simulink model "AirCraft_Fuel_Distribution"  (R2023b)
settings: Solver=VariableStepAuto  StartTime=0.0  StopTime=8000  MaxStep=10  RelTol=1e-04  AbsTol=1e-04
undefined symbols (not defined in the file): cutoff_time_const, mover_time_constant, opening_max, pump_engine, pump_wing, rho_ref, vol_fuel_min
libraries: fl_lib x52, nesl_utility x33, SimscapeFluids_lib x17, simulink_extras x11, SignalEditorBlockLib x2
(part 1 of 2)
settings Model: Creator=Asus
settings SolverCC: MaxConsecutiveMinStep=4  ZeroCrossAlgorithm=Adaptive  AlgebraicLoopSolver=LineSearch
settings DebuggingCC: AlgebraicLoopMsg=none  IgnoredZcDiagnostic=none  UnconnectedInputMsg=warning  UnconnectedOutputMsg=warning  UnconnectedLineMsg=warning
settings ModelReferenceCC: EnableRefExpFcnMdlSchedulingChecks=on

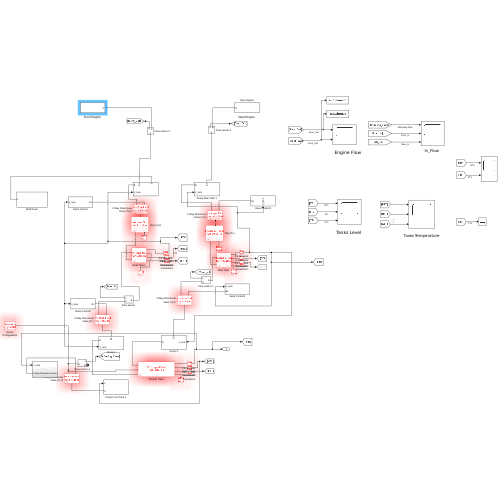
[thumbnail: Simulink's stored preview of the top-level diagram]
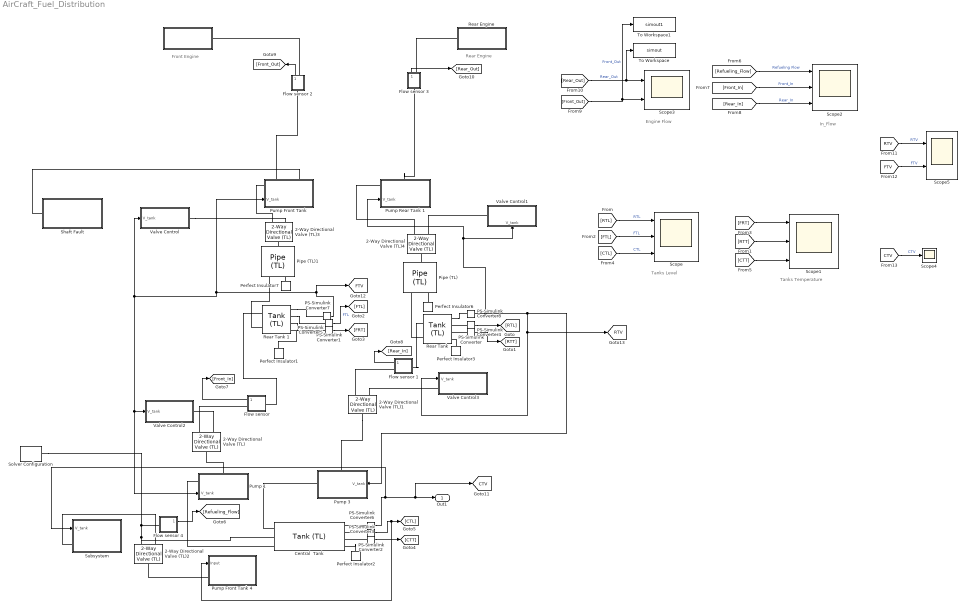
== system AirCraft_Fuel_Distribution ==
  note: Front Engine
  note: Rear Engine
  note: Tanks Temperature
  note: Tanks Level
  note: In_Flow
  note: Engine Flow
  " " : Subsystem
  2-Way Directional Valve (TL) : SimscapeFluids_lib/Thermal Liquid/Valves & Orifices/Directional Control Valves/2-Way Directional Valve (TL)  valve_spec=fluids.thermal_liquid.valves.enum.orifice_spec.linear  opening_max=opening_max m  area_max=area_max m^2  area_leak=1e-10 m^2  smoothing_factor=0.01  opening_TLU=[-.002, 0, .002, .005, .015] m  valve_area_TLU=[1e-09, 2.0352e-07, 4.0736e-05, .00011438, .00034356] m^2  Cd=0.7  Re_c=12  opening_mdot_TLU=[-.002, 0, .002, .005, .015] m  p_diff_TLU=[-.1, .3, .5, .7] MPa  mdot_TLU=[-1e-05, 1.7e-05, 2e-05, 2.6e-05; -.002, .0035, .0045, .0053; -.4, .7, .9, 1.06; -1.13, 1.96, 2.5, 3; -3.45, 6, 7.7, 9.13] kg/s  T_ref_in=293.15 K  p_ref_in=0.101325 MPa  x0=area_max m  area=0.001 m^2  length=0.1 m
      settings: InternalSimscapePortConfiguration="{\"Bottom\":[],\"Left\":[{\"id\":\"A\",\"label\":\"A\",\"type\":\"foundation.thermal_liquid.thermal_liquid\"}],\"Right\":[{\"id\":\"S\",\"label\":\"S\",\"type\":\"input\"},{\"id\":\"B\",\"label\":\"B\",\"type\":\"foundation.thermal_liquid.thermal_liquid\"}],\"Top\":[]}"
  2-Way Directional Valve (TL)1 : SimscapeFluids_lib/Thermal Liquid/Valves & Orifices/Directional Control Valves/2-Way Directional Valve (TL)  valve_spec=fluids.thermal_liquid.valves.enum.orifice_spec.linear  opening_max=opening_max m  area_max=area_max m^2  area_leak=1e-10 m^2  smoothing_factor=0.01  opening_TLU=[-.002, 0, .002, .005, .015] m  valve_area_TLU=[1e-09, 2.0352e-07, 4.0736e-05, .00011438, .00034356] m^2  Cd=0.7  Re_c=12  opening_mdot_TLU=[-.002, 0, .002, .005, .015] m  p_diff_TLU=[-.1, .3, .5, .7] MPa  mdot_TLU=[-1e-05, 1.7e-05, 2e-05, 2.6e-05; -.002, .0035, .0045, .0053; -.4, .7, .9, 1.06; -1.13, 1.96, 2.5, 3; -3.45, 6, 7.7, 9.13] kg/s  T_ref_in=293.15 K  p_ref_in=0.101325 MPa  x0=opening_max m  area=0.001 m^2  length=0.1 m
      settings: InternalSimscapePortConfiguration="{\"Bottom\":[],\"Left\":[{\"id\":\"A\",\"label\":\"A\",\"type\":\"foundation.thermal_liquid.thermal_liquid\"}],\"Right\":[{\"id\":\"S\",\"label\":\"S\",\"type\":\"input\"},{\"id\":\"B\",\"label\":\"B\",\"type\":\"foundation.thermal_liquid.thermal_liquid\"}],\"Top\":[]}"
  2-Way Directional Valve (TL)2 : SimscapeFluids_lib/Thermal Liquid/Valves & Orifices/Directional Control Valves/2-Way Directional Valve (TL)  valve_spec=fluids.thermal_liquid.valves.enum.orifice_spec.linear  opening_max=opening_max m  area_max=area_max m^2  area_leak=1e-10 m^2  smoothing_factor=0.01  opening_TLU=[-.002, 0, .002, .005, .015] m  valve_area_TLU=[1e-09, 2.0352e-07, 4.0736e-05, .00011438, .00034356] m^2  Cd=0.7  Re_c=12  opening_mdot_TLU=[-.002, 0, .002, .005, .015] m  p_diff_TLU=[-.1, .3, .5, .7] MPa  mdot_TLU=[-1e-05, 1.7e-05, 2e-05, 2.6e-05; -.002, .0035, .0045, .0053; -.4, .7, .9, 1.06; -1.13, 1.96, 2.5, 3; -3.45, 6, 7.7, 9.13] kg/s  T_ref_in=293.15 K  p_ref_in=0.101325 MPa  x0=area_max m  area=0.001 m^2  length=0.1 m
      settings: InternalSimscapePortConfiguration="{\"Bottom\":[],\"Left\":[{\"id\":\"A\",\"label\":\"A\",\"type\":\"foundation.thermal_liquid.thermal_liquid\"}],\"Right\":[{\"id\":\"S\",\"label\":\"S\",\"type\":\"input\"},{\"id\":\"B\",\"label\":\"B\",\"type\":\"foundation.thermal_liquid.thermal_liquid\"}],\"Top\":[]}"
  2-Way Directional Valve (TL)3 : SimscapeFluids_lib/Thermal Liquid/Valves & Orifices/Directional Control Valves/2-Way Directional Valve (TL)  valve_spec=fluids.thermal_liquid.valves.enum.orifice_spec.linear  opening_max=opening_max m  area_max=area_max m^2  area_leak=1e-10 m^2  smoothing_factor=0.01  opening_TLU=[-.002, 0, .002, .005, .015] m  valve_area_TLU=[1e-09, 2.0352e-07, 4.0736e-05, .00011438, .00034356] m^2  Cd=0.7  Re_c=12  opening_mdot_TLU=[-.002, 0, .002, .005, .015] m  p_diff_TLU=[-.1, .3, .5, .7] MPa  mdot_TLU=[-1e-05, 1.7e-05, 2e-05, 2.6e-05; -.002, .0035, .0045, .0053; -.4, .7, .9, 1.06; -1.13, 1.96, 2.5, 3; -3.45, 6, 7.7, 9.13] kg/s  T_ref_in=293.15 K  p_ref_in=0.101325 MPa  x0=opening_max m  area=0.001 m^2  length=0.1 m
      settings: InternalSimscapePortConfiguration="{\"Bottom\":[],\"Left\":[{\"id\":\"A\",\"label\":\"A\",\"type\":\"foundation.thermal_liquid.thermal_liquid\"}],\"Right\":[{\"id\":\"S\",\"label\":\"S\",\"type\":\"input\"},{\"id\":\"B\",\"label\":\"B\",\"type\":\"foundation.thermal_liquid.thermal_liquid\"}],\"Top\":[]}"
  2-Way Directional Valve (TL)4 : SimscapeFluids_lib/Thermal Liquid/Valves & Orifices/Directional Control Valves/2-Way Directional Valve (TL)  valve_spec=fluids.thermal_liquid.valves.enum.orifice_spec.linear  opening_max=opening_max m  area_max=area_max m^2  area_leak=1e-10 m^2  smoothing_factor=0.01  opening_TLU=[-.002, 0, .002, .005, .015] m  valve_area_TLU=[1e-09, 2.0352e-07, 4.0736e-05, .00011438, .00034356] m^2  Cd=0.7  Re_c=12  opening_mdot_TLU=[-.002, 0, .002, .005, .015] m  p_diff_TLU=[-.1, .3, .5, .7] MPa  mdot_TLU=[-1e-05, 1.7e-05, 2e-05, 2.6e-05; -.002, .0035, .0045, .0053; -.4, .7, .9, 1.06; -1.13, 1.96, 2.5, 3; -3.45, 6, 7.7, 9.13] kg/s  T_ref_in=293.15 K  p_ref_in=0.101325 MPa  x0=opening_max m  area=0.001 m^2  length=0.1 m
      settings: InternalSimscapePortConfiguration="{\"Bottom\":[],\"Left\":[{\"id\":\"A\",\"label\":\"A\",\"type\":\"foundation.thermal_liquid.thermal_liquid\"}],\"Right\":[{\"id\":\"S\",\"label\":\"S\",\"type\":\"input\"},{\"id\":\"B\",\"label\":\"B\",\"type\":\"foundation.thermal_liquid.thermal_liquid\"}],\"Top\":[]}"
  "Central  Tank " : SimscapeFluids_lib/Thermal Liquid/Tanks & Accumulators/Tank (TL)  pressure_spec=2  tank_pressure=p_tank MPa  max_capacity=384 m^3  volume_spec=2  tank_area=center_tank_level_TLU m^2  level_TLU=center_tank_level_TLU m  volume_TLU=center_tank_volume_TLU m^3  inlet_height=0.1 m  inlet_area=0.01 m^2  g=9.81 m/s^2  level_specify=on  level_priority=High  level=0.5 m  level_nominal_specify=off  level_nominal_unit=m  level_nominal_value=1  volume_specify=on  volume_priority=None  volume=3 m^3  volume_nominal_specify=off  volume_nominal_unit=m^3  volume_nominal_value=1  mass_specify=off  mass_priority=None  mass=5e+3 kg  mass_nominal_specify=off  mass_nominal_unit=kg  mass_nominal_value=1  T_tank_specify=on  T_tank_priority=High  T_tank=T0 K  T_tank_nominal_specify=off  T_tank_nominal_unit=K  T_tank_nominal_value=1  inlet_heights_AB=[.1, 0] m  inlet_areas_AB=[.01, .01] m^2  inlet_heights_ABC=[1e-4, 1e-4, 0] m  inlet_areas_ABC=7e-4 .* ones(1,3) m^2
      settings: InternalSimscapePortConfiguration="{\"Bottom\":[],\"Left\":[{\"id\":\"A\",\"label\":\"A\",\"type\":\"foundation.thermal_liquid.thermal_liquid\"},{\"id\":\"B\",\"label\":\"B\",\"type\":\"foundation.thermal_liquid.thermal_liquid\"},{\"id\":\"C\",\"label\":\"C\",\"type\":\"foundation.thermal_liquid.thermal_liquid\"}],\"Right\":[{\"id\":\"V_out\",\"label\":\"V\",\"type\":\"output\"},{\"id\":\"L_out\",\"label\":\"L\",\"type\":\"output\"},{\"id\":\"T_out\",\"label\":\"T\",\"type\":\"output\"},{\"id\":\"H\",\"label\":\"H\",\"type\":\"foundation.thermal.thermal\"}],\"Top\":[]}"
  "Flow sensor " : Subsystem
      settings: PortSchema="{\"entries\":[{\"content\":{\"sides\":[{\"content\":{\"connectorIds\":[\"Out1\",\"LConn1\"]},\"type\":\"ConnectorPlacement.EquallySpacedRectSide\",\"uuid\":\"5284a614-22fb-4539-b8c2-000aa98607e7\"},{\"content\":{\"connectorIds\":[\"RConn1\"],\"side\":\"RIGHT\"},\"type\":\"ConnectorPlacement.EquallySpacedRectSide\",\"uuid\":\"ab54947e-968b-43fc-9d3b-310523b757f2\"},{\"content\":{\"connectorIds\":[],\"side\":\"TOP\"},\"type\":\"ConnectorPlacement.EquallySpacedRectSide\",\"uuid\":\"346eb7b4-d6d4-447e-a1ee-2e30abc93d9f\"}]},\"type\":\"ConnectorPlacement.EquallySpacedConnector\",\"uuid\":\"c574b111-9014-4fd2-84a0-cd6807004c01\"}],\"packageUris\":[\"http://schema.mathworks.com/mf0/Connector/19700101\"],\"version\":\"1.0\"}"
  Flow sensor 1 : Subsystem
      settings: PortSchema="{\"entries\":[{\"content\":{\"sides\":[{\"content\":{\"connectorIds\":[\"Out1\",\"LConn1\"]},\"type\":\"ConnectorPlacement.EquallySpacedRectSide\",\"uuid\":\"5284a614-22fb-4539-b8c2-000aa98607e7\"},{\"content\":{\"connectorIds\":[\"RConn1\"],\"side\":\"RIGHT\"},\"type\":\"ConnectorPlacement.EquallySpacedRectSide\",\"uuid\":\"ab54947e-968b-43fc-9d3b-310523b757f2\"},{\"content\":{\"connectorIds\":[],\"side\":\"TOP\"},\"type\":\"ConnectorPlacement.EquallySpacedRectSide\",\"uuid\":\"346eb7b4-d6d4-447e-a1ee-2e30abc93d9f\"}]},\"type\":\"ConnectorPlacement.EquallySpacedConnector\",\"uuid\":\"c574b111-9014-4fd2-84a0-cd6807004c01\"}],\"packageUris\":[\"http://schema.mathworks.com/mf0/Connector/19700101\"],\"version\":\"1.0\"}"
  Flow sensor 2 : Subsystem
  Flow sensor 3 : Subsystem
  Flow sensor 4 : Subsystem
  PS-Simulink Converter{,1..8} (9 alike) : nesl_utility/PS-Simulink Converter  PhysicalDomain=network_engine_domain  SubClassName=ps_output  LeftPortType=input  RightPortType=output  PseudoPeriodic=off  Frequencies=[]  Unit=inherit  AffineConversion=off
  Perfect Insulator{1..3,6..7} (5 alike) : fl_lib/Thermal/Thermal Elements/Perfect Insulator  T_specify=off  T_priority=None  T=0 K  T_nominal_specify=off  T_nominal_unit=K  T_nominal_value=1
  Pipe (TL) : SimscapeFluids_lib/Thermal Liquid/Pipes & Fittings/Pipe (TL)  dynamic_compressibility=1  inertia=0  num_segments=1  pipe_length=1 m  area=0.001 m^2  Dh=0.1128 m  wall_spec=1  Dh_rigid=0.0254 m  wall_compliance=1.2e-6 m/MPa  wall_time_constant=0.01 s  elevation_gain=0 m  g=9.81 m/s^2  pressure_loss_spec=1  length_add=1 m  roughness=1.5e-5 m  Re_friction_TLU=[ 400 1000 1.5e+3 3e+3 4e+3 6e+3 1e+4 2e+4 4e+4 6e+4 1e+5 1e+8 ]  friction_factor_TLU=[ 0.264 0.112 0.07099999999999999 0.0417 0.0387 0.0268 0.025 0.0232 0.0226 0.022 0.0214 0.0214 ]  shape_factor=64  mdot_nominal=[ 0.1 1 ] kg/s  p_diff_nominal=[ 0.001 0.01 ] MPa  mdot_threshold=1e-6 kg/s  Re_lam=2e+3  Re_tur=4e+3  heat_transfer_spec=1  mdot_nominal_heat=[ 0.1 1 ] kg/s  T_in_nominal=[ 293.15 293.15 ] K  T_out_nominal=[ 300 300 ] K  p_in_nominal_heat=[ 0.101325 0.101325 ] MPa  T_wall_nominal=[ 303.15 303.15 ] K  a_coeff=0.023  b_Re_power=0.8  c_Pr_power=0.4  Nu_lam=3.66  Re_Colburn_TLU=[ 100 150 1000 ]  Colburn_factor_TLU=[ 0.019 0.013 0.002 ]  Re_Nu_TLU=[ 100 150 1000 ]  Pr_Nu_TLU=[ 1 10 ]  Nu_TLU=[ 3.72 4.21; 3.75 4.44; 4.21 7.15 ]  T0_vec=T0 K  p0_vec=p0 MPa  mdot0=0.1 kg/s
  Pipe (TL)1 : SimscapeFluids_lib/Thermal Liquid/Pipes & Fittings/Pipe (TL)  dynamic_compressibility=1  inertia=0  num_segments=1  pipe_length=1 m  area=0.001 m^2  Dh=0.1128 m  wall_spec=1  Dh_rigid=0.0254 m  wall_compliance=1.2e-6 m/MPa  wall_time_constant=0.01 s  elevation_gain=0 m  g=9.81 m/s^2  pressure_loss_spec=1  length_add=1 m  roughness=1.5e-5 m  Re_friction_TLU=[ 400 1000 1.5e+3 3e+3 4e+3 6e+3 1e+4 2e+4 4e+4 6e+4 1e+5 1e+8 ]  friction_factor_TLU=[ 0.264 0.112 0.07099999999999999 0.0417 0.0387 0.0268 0.025 0.0232 0.0226 0.022 0.0214 0.0214 ]  shape_factor=64  mdot_nominal=[ 0.1 1 ] kg/s  p_diff_nominal=[ 0.001 0.01 ] MPa  mdot_threshold=1e-6 kg/s  Re_lam=2e+3  Re_tur=4e+3  heat_transfer_spec=1  mdot_nominal_heat=[ 0.1 1 ] kg/s  T_in_nominal=[ 293.15 293.15 ] K  T_out_nominal=[ 300 300 ] K  p_in_nominal_heat=[ 0.101325 0.101325 ] MPa  T_wall_nominal=[ 303.15 303.15 ] K  a_coeff=0.023  b_Re_power=0.8  c_Pr_power=0.4  Nu_lam=3.66  Re_Colburn_TLU=[ 100 150 1000 ]  Colburn_factor_TLU=[ 0.019 0.013 0.002 ]  Re_Nu_TLU=[ 100 150 1000 ]  Pr_Nu_TLU=[ 1 10 ]  Nu_TLU=[ 3.72 4.21; 3.75 4.44; 4.21 7.15 ]  T0_vec=T0 K  p0_vec=p0 MPa  mdot0=0.1 kg/s
  Pump 1 : Subsystem
      settings: PortSchema="{\"entries\":[{\"content\":{\"sides\":[{\"content\":{\"connectorIds\":[\"LConn1\",\"In1\"]},\"type\":\"ConnectorPlacement.EquallySpacedRectSide\",\"uuid\":\"f9fde711-b4bf-4785-9cc0-8903af8b3bdb\"},{\"content\":{\"connectorIds\":[],\"side\":\"RIGHT\"},\"type\":\"ConnectorPlacement.EquallySpacedRectSide\",\"uuid\":\"7d5e19b5-7f0d-4770-805b-c0a3bf695392\"},{\"content\":{\"connectorIds\":[\"LConn2\"],\"side\":\"TOP\"},\"type\":\"ConnectorPlacement.EquallySpacedRectSide\",\"uuid\":\"e5badb16-c1b0-4e24-af75-188c6a2d2ae0\"},{\"content\":{\"connectorIds\":[],\"side\":\"BOTTOM\"},\"type\":\"ConnectorPlacement.EquallySpacedRectSide\",\"uuid\":\"d755c16a-0870-4c35-a487-3c7ff45286b1\"}]},\"type\":\"ConnectorPlacement.EquallySpacedConnector\",\"uuid\":\"e7d75403-c0b4-4ff8-841b-0a077d0a7f1c\"}],\"packageUris\":[\"http://schema.mathworks.com/mf0/Connector/19700101\"],\"version\":\"1.0\"}"
  Pump 3 : Subsystem
      settings: PortSchema="{\"entries\":[{\"content\":{\"sides\":[{\"content\":{\"connectorIds\":[\"LConn1\"]},\"type\":\"ConnectorPlacement.EquallySpacedRectSide\",\"uuid\":\"f9fde711-b4bf-4785-9cc0-8903af8b3bdb\"},{\"content\":{\"connectorIds\":[\"In1\"],\"side\":\"RIGHT\"},\"type\":\"ConnectorPlacement.EquallySpacedRectSide\",\"uuid\":\"7d5e19b5-7f0d-4770-805b-c0a3bf695392\"},{\"content\":{\"connectorIds\":[\"LConn2\"],\"side\":\"TOP\"},\"type\":\"ConnectorPlacement.EquallySpacedRectSide\",\"uuid\":\"e5badb16-c1b0-4e24-af75-188c6a2d2ae0\"},{\"content\":{\"connectorIds\":[],\"side\":\"BOTTOM\"},\"type\":\"ConnectorPlacement.EquallySpacedRectSide\",\"uuid\":\"d755c16a-0870-4c35-a487-3c7ff45286b1\"}]},\"type\":\"ConnectorPlacement.EquallySpacedConnector\",\"uuid\":\"e7d75403-c0b4-4ff8-841b-0a077d0a7f1c\"}],\"packageUris\":[\"http://schema.mathworks.com/mf0/Connector/19700101\"],\"version\":\"1.0\"}"
  "Pump Front Tank " : Subsystem
      settings: PortSchema="{\"entries\":[{\"content\":{\"sides\":[{\"content\":{\"connectorIds\":[\"LConn1\",\"In1\"]},\"type\":\"ConnectorPlacement.EquallySpacedRectSide\",\"uuid\":\"f9fde711-b4bf-4785-9cc0-8903af8b3bdb\"},{\"content\":{\"connectorIds\":[],\"side\":\"RIGHT\"},\"type\":\"ConnectorPlacement.EquallySpacedRectSide\",\"uuid\":\"7d5e19b5-7f0d-4770-805b-c0a3bf695392\"},{\"content\":{\"connectorIds\":[\"LConn2\",\"LConn3\"],\"side\":\"TOP\"},\"type\":\"ConnectorPlacement.EquallySpacedRectSide\",\"uuid\":\"e5badb16-c1b0-4e24-af75-188c6a2d2ae0\"},{\"content\":{\"connectorIds\":[],\"side\":\"BOTTOM\"},\"type\":\"ConnectorPlacement.EquallySpacedRectSide\",\"uuid\":\"d755c16a-0870-4c35-a487-3c7ff45286b1\"}]},\"type\":\"ConnectorPlacement.EquallySpacedConnector\",\"uuid\":\"e7d75403-c0b4-4ff8-841b-0a077d0a7f1c\"}],\"packageUris\":[\"http://schema.mathworks.com/mf0/Connector/19700101\"],\"version\":\"1.0\"}"
  Pump Front Tank 4 : Subsystem
  Pump Rear Tank 1 : Subsystem
      settings: PortSchema="{\"entries\":[{\"content\":{\"sides\":[{\"content\":{\"connectorIds\":[\"LConn1\",\"In1\"]},\"type\":\"ConnectorPlacement.EquallySpacedRectSide\",\"uuid\":\"f9fde711-b4bf-4785-9cc0-8903af8b3bdb\"},{\"content\":{\"connectorIds\":[],\"side\":\"RIGHT\"},\"type\":\"ConnectorPlacement.EquallySpacedRectSide\",\"uuid\":\"7d5e19b5-7f0d-4770-805b-c0a3bf695392\"},{\"content\":{\"connectorIds\":[\"LConn2\"],\"side\":\"TOP\"},\"type\":\"ConnectorPlacement.EquallySpacedRectSide\",\"uuid\":\"e5badb16-c1b0-4e24-af75-188c6a2d2ae0\"},{\"content\":{\"connectorIds\":[],\"side\":\"BOTTOM\"},\"type\":\"ConnectorPlacement.EquallySpacedRectSide\",\"uuid\":\"d755c16a-0870-4c35-a487-3c7ff45286b1\"}]},\"type\":\"ConnectorPlacement.EquallySpacedConnector\",\"uuid\":\"e7d75403-c0b4-4ff8-841b-0a077d0a7f1c\"}],\"packageUris\":[\"http://schema.mathworks.com/mf0/Connector/19700101\"],\"version\":\"1.0\"}"
  Rear Engine : Subsystem
  "Rear Tank " : SimscapeFluids_lib/Thermal Liquid/Tanks & Accumulators/Tank (TL)  pressure_spec=2  tank_pressure=p_tank MPa  max_capacity=12 m^3  volume_spec=2  tank_area=1 m^2  level_TLU=wing_tank_level_TLU m  volume_TLU=wing_tank_volume_TLU m^3  inlet_height=0.1 m  inlet_area=0.01 m^2  g=9.81 m/s^2  level_specify=off  level_priority=High  level=5 m  level_nominal_specify=off  level_nominal_unit=m  level_nominal_value=1  volume_specify=on  volume_priority=None  volume=10 m^3  volume_nominal_specify=off  volume_nominal_unit=m^3  volume_nominal_value=1  mass_specify=off  mass_priority=None  mass=5e+3 kg  mass_nominal_specify=off  mass_nominal_unit=kg  mass_nominal_value=1  T_tank_specify=on  T_tank_priority=High  T_tank=T0 K  T_tank_nominal_specify=off  T_tank_nominal_unit=K  T_tank_nominal_value=1  inlet_heights_AB=[0, 0] m  inlet_areas_AB=[.001, .001] m^2  inlet_heights_ABC=[.1, .05, 0] m  inlet_areas_ABC=[.01, .01, .01] m^2
      settings: InternalSimscapePortConfiguration="{\"Bottom\":[],\"Left\":[{\"id\":\"A\",\"label\":\"A\",\"type\":\"foundation.thermal_liquid.thermal_liquid\"},{\"id\":\"B\",\"label\":\"B\",\"type\":\"foundation.thermal_liquid.thermal_liquid\"}],\"Right\":[{\"id\":\"V_out\",\"label\":\"V\",\"type\":\"output\"},{\"id\":\"L_out\",\"label\":\"L\",\"type\":\"output\"},{\"id\":\"T_out\",\"label\":\"T\",\"type\":\"output\"},{\"id\":\"H\",\"label\":\"H\",\"type\":\"foundation.thermal.thermal\"}],\"Top\":[]}"
  Rear Tank 1 : SimscapeFluids_lib/Thermal Liquid/Tanks & Accumulators/Tank (TL)  pressure_spec=2  tank_pressure=p_tank MPa  max_capacity=12 m^3  volume_spec=2  tank_area=1 m^2  level_TLU=wing_tank_level_TLU m  volume_TLU=wing_tank_volume_TLU m^3  inlet_height=0.1 m  inlet_area=0.01 m^2  g=9.81 m/s^2  level_specify=off  level_priority=High  level=5 m  level_nominal_specify=off  level_nominal_unit=m  level_nominal_value=1  volume_specify=on  volume_priority=None  volume=10 m^3  volume_nominal_specify=off  volume_nominal_unit=m^3  volume_nominal_value=1  mass_specify=off  mass_priority=None  mass=5e+3 kg  mass_nominal_specify=off  mass_nominal_unit=kg  mass_nominal_value=1  T_tank_specify=on  T_tank_priority=High  T_tank=T0 K  T_tank_nominal_specify=off  T_tank_nominal_unit=K  T_tank_nominal_value=1  inlet_heights_AB=[0, 0] m  inlet_areas_AB=[.001, .001] m^2  inlet_heights_ABC=[.1, .05, 0] m  inlet_areas_ABC=[.01, .01, .01] m^2
      settings: InternalSimscapePortConfiguration="{\"Bottom\":[],\"Left\":[{\"id\":\"A\",\"label\":\"A\",\"type\":\"foundation.thermal_liquid.thermal_liquid\"},{\"id\":\"B\",\"label\":\"B\",\"type\":\"foundation.thermal_liquid.thermal_liquid\"}],\"Right\":[{\"id\":\"V_out\",\"label\":\"V\",\"type\":\"output\"},{\"id\":\"L_out\",\"label\":\"L\",\"type\":\"output\"},{\"id\":\"T_out\",\"label\":\"T\",\"type\":\"output\"},{\"id\":\"H\",\"label\":\"H\",\"type\":\"foundation.thermal.thermal\"}],\"Top\":[]}"
  Scope : Scope  NumInputPorts=3
  Scope1 : Scope  NumInputPorts=3
  Scope2 : Scope  NumInputPorts=3
  Scope3 : Scope  NumInputPorts=2
  Scope4 : Scope
  Scope5 : Scope  NumInputPorts=2
  "Shaft Fault " : Subsystem
  Solver Configuration : nesl_utility/Solver Configuration  PhysicalDomain=network_engine_domain  SubClassName=solver  LeftPortType=input  RightPortType=generic  Tones=[]  Harmonics=[]  SimulateNoise=off  Profile=off  UseLocalSampling=off  EnableSwitchedLinearOptims=on  FrequencyDomain=off  UseCCode=off  RelTol=0.001  AbsTol=1e-06  MinStep=1e-09  ToWorkspace=off  RevertToSquareIcSolve=off  NumHomotopyIterations=100  PhasorMode=off  PhasorModeNumHarmonics=1  DoDC=off  ResidualTolerance=1e-09  UseLocalSolver=off  LocalSolverChoice=NE_BACKWARD_EULER_ADVANCER  LocalSolverSampleTime=0.001  DoFixedCost=off  MaxNonlinIter=3  MaxModeIter=2  LinearAlgebra=auto  EquationFormulation=NE_TIME_EF  DelaysMemoryBudget=1024  AutomaticFiltering=on  FilteringTimeConstant=0.001  PartitionStorageMethod=AS_NEEDED  PartitionMemoryBudget=1024  PartitionMethod=ROBUST
  Subsystem : Subsystem
  To Workspace : ToWorkspace  VariableName=simout  SaveFormat=Timeseries  SampleTime=-1
  To Workspace1 : ToWorkspace  VariableName=simout1  SaveFormat=Timeseries  SampleTime=-1
  Valve Control : Subsystem
  Valve Control1 : Subsystem
      settings: PortSchema="{\"entries\":[{\"content\":{\"sides\":[{\"content\":{\"connectorIds\":[\"LConn1\"]},\"type\":\"ConnectorPlacement.EquallySpacedRectSide\",\"uuid\":\"5ad770cd-1604-404c-96fd-b2e6ab98ce29\"},{\"content\":{\"connectorIds\":[],\"side\":\"RIGHT\"},\"type\":\"ConnectorPlacement.EquallySpacedRectSide\",\"uuid\":\"be0e744c-dbb3-4b13-9c18-b642da714a48\"},{\"content\":{\"connectorIds\":[],\"side\":\"TOP\"},\"type\":\"ConnectorPlacement.EquallySpacedRectSide\",\"uuid\":\"703d76ce-9870-4037-95ca-3762ac4fc19e\"},{\"content\":{\"connectorIds\":[\"In1\"],\"side\":\"BOTTOM\"},\"type\":\"ConnectorPlacement.EquallySpacedRectSide\",\"uuid\":\"43b1032c-5275-45be-bae5-4565a523b82a\"}]},\"type\":\"ConnectorPlacement.EquallySpacedConnector\",\"uuid\":\"80c43ebb-b9de-4469-a8c7-4b83e80440f3\"}],\"packageUris\":[\"http://schema.mathworks.com/mf0/Connector/19700101\"],\"version\":\"1.0\"}"
  Valve Control2 : Subsystem
  Valve Control3 : Subsystem
  Out1 : Outport
  tag scope: CTV=global, FTV=global, RTV=global
  wires:
  PS-Simulink Converter/1 -> [RTL]
  PS-Simulink Converter4/1 -> [RTT]
  [RTL] -> Scope/1  "RTL"
  [RTT] -> Scope1/2
  PS-Simulink Converter1/1 -> [FTL]  "FTL"
  PS-Simulink Converter5/1 -> [FRT]
  [FRT] -> Scope1/1
  [FTL] -> Scope/2  "FTL"
  PS-Simulink Converter2/1 -> Pump Front Tank 4/1(Input), [CTL]
  PS-Simulink Converter3/1 -> [CTT]
  [CTL] -> Scope/3  "CTL"
  [CTT] -> Scope1/3
  Flow sensor 4/1(Out1) -> [Refueling_Flow]
  "Flow sensor "/1(Out1) -> [Front_In]
  Flow sensor 1/1(Out1) -> [Rear_In]
  [Front_In] -> Scope2/2  "Front_In"
  [Refueling_Flow] -> Scope2/1  "Refueling Flow"
  [Rear_In] -> Scope2/3  "Rear_In"
  Flow sensor 2/1(Out1) -> [Front_Out]
  Flow sensor 3/1(Out1) -> [Rear_Out]
  [Rear_Out] -> To Workspace/1, Scope3/1  "Rear_Out"
  [Front_Out] -> To Workspace1/1, Scope3/2  "Front_Out"
  PS-Simulink Converter6/1 -> Subsystem/1(V_tank), [CTV], Out1/1
  PS-Simulink Converter7/1 -> Valve Control/1(V_tank), Valve Control2/1(V_tank), Pump 1/1(V_tank), "Pump Front Tank "/1(V_tank), [FTV]
  PS-Simulink Converter8/1 -> Pump 3/1(V_tank), [RTV], Valve Control3/1(V_tank), Pump Rear Tank 1/1(V_tank), Valve Control1/1(V_tank)
  [RTV] -> Scope5/1  "RTV"
  [FTV] -> Scope5/2  "FTV"
  [CTV] -> Scope4/1  "CTV"
  connections:
  Perfect Insulator3/LConn1 -- "Rear Tank "/RConn4
  Perfect Insulator2/LConn1 -- "Central  Tank "/RConn4
  PS-Simulink Converter/LConn1 -- "Rear Tank "/RConn2
  PS-Simulink Converter2/LConn1 -- "Central  Tank "/RConn2
  PS-Simulink Converter3/LConn1 -- "Central  Tank "/RConn3
  PS-Simulink Converter4/LConn1 -- "Rear Tank "/RConn3
  Valve Control/RConn1 -- 2-Way Directional Valve (TL)3/RConn1
  2-Way Directional Valve (TL)4/RConn1 -- Valve Control1/LConn1
  Valve Control2/RConn1 -- 2-Way Directional Valve (TL)/RConn1
  2-Way Directional Valve (TL)1/RConn1 -- Valve Control3/LConn1
  PS-Simulink Converter6/LConn1 -- "Central  Tank "/RConn1
  "Rear Tank "/RConn1 -- PS-Simulink Converter8/LConn1
  Pump Front Tank 4/LConn1 -- 2-Way Directional Valve (TL)2/LConn1
  2-Way Directional Valve (TL)2/RConn2 -- "Central  Tank "/LConn2 -- Solver Configuration/RConn1 -- Flow sensor 4/LConn1
  Subsystem/LConn1 -- 2-Way Directional Valve (TL)2/RConn1
  Flow sensor 1/RConn1 -- "Rear Tank "/LConn1
  Pump 1/LConn2 -- 2-Way Directional Valve (TL)/LConn1
  2-Way Directional Valve (TL)/RConn2 -- "Flow sensor "/LConn1
  2-Way Directional Valve (TL)1/LConn1 -- Pump 3/LConn2
  2-Way Directional Valve (TL)1/RConn2 -- Flow sensor 1/LConn1
  2-Way Directional Valve (TL)3/RConn2 -- "Pump Front Tank "/LConn1
  2-Way Directional Valve (TL)4/RConn2 -- Pump Rear Tank 1/LConn1
  "Central  Tank "/LConn3 -- Pump 1/LConn1
  "Central  Tank "/LConn1 -- Pump 3/LConn1
  Flow sensor 2/RConn1 -- " "/RConn1
  Flow sensor 3/RConn1 -- Rear Engine/RConn1
  Pipe (TL)/RConn1 -- 2-Way Directional Valve (TL)4/LConn1
  "Rear Tank "/LConn2 -- Pipe (TL)/LConn1
  Perfect Insulator6/LConn1 -- Pipe (TL)/LConn2
  Pipe (TL)1/RConn1 -- 2-Way Directional Valve (TL)3/LConn1
  Perfect Insulator7/LConn1 -- Pipe (TL)1/LConn2
  "Pump Front Tank "/LConn2 -- Flow sensor 2/LConn1
  Pump Rear Tank 1/LConn2 -- Flow sensor 3/LConn1
  Rear Tank 1/LConn1 -- "Flow sensor "/RConn1
  Rear Tank 1/LConn2 -- Pipe (TL)1/LConn1
  Rear Tank 1/RConn1 -- PS-Simulink Converter7/LConn1
  Rear Tank 1/RConn2 -- PS-Simulink Converter1/LConn1
  Rear Tank 1/RConn3 -- PS-Simulink Converter5/LConn1
  Perfect Insulator1/LConn1 -- Rear Tank 1/RConn4
  "Shaft Fault "/LConn1 -- "Pump Front Tank "/LConn3

== system AirCraft_Fuel_Distribution/  ==
  Centrifugal Pump (TL) : SimscapeFluids_lib/Thermal Liquid/Pumps & Motors/Centrifugal Pump (TL)  pump_parameterization=2  mech_orientation=1  flow_rate_1D_TLU=[16.67, 30, 40, 53.33, 66.67, 83.33] lpm  head_1D_TLU=[50, 47.5, 45, 40, 35, 25] m  power_1D_TLU=[.6, .75, .85, .93, .98, .99] kW  rho_ref_1D=998 kg/m^3  omega_ref_1D=3500 rpm  flow_rate_2D_TLU=[16.67, 23.33, 30, 40, 53.33, 60] lpm  omega_2D_TLU=[2450, 2800, 3150, 3500] rpm  head_2D_TLU=[25, 32.7, 42.5, 50; 24, 31.7, 41, 49; 22.7, 30.5, 39, 47.5; 20, 28, 36, 45; 15.7, 24, 32, 40; 12.5, 21, 29.5, 37.5] m  power_2D_TLU=[.28, .38, .5, .6; .31, .41, .55, .68; .33, .44, .6, .75; .36, .48, .65, .83; .38, .53, .72, .93; .39, .55, .75, .97] kW  rho_ref_2D=920 kg/m^3  omega_threshold=10 rad/s  area=0.01 m^2  mdot_A_specify=off  mdot_A_priority=None  mdot_A=1 kg/s  mdot_A_nominal_specify=off  mdot_A_nominal_unit=kg/s  mdot_A_nominal_value=1
      settings: InternalSimscapePortConfiguration="{\"Bottom\":[],\"Left\":[{\"id\":\"A\",\"label\":\"A\",\"type\":\"foundation.thermal_liquid.thermal_liquid\"},{\"id\":\"B\",\"label\":\"B\",\"type\":\"foundation.thermal_liquid.thermal_liquid\"}],\"Right\":[{\"id\":\"R\",\"label\":\"R\",\"type\":\"foundation.mechanical.rotational.rotational\"},{\"id\":\"C\",\"label\":\"C\",\"type\":\"foundation.mechanical.rotational.rotational\"}],\"Top\":[]}"
  Ideal Angular Velocity Source2 : fl_lib/Mechanical/Mechanical Sources/Ideal Angular Velocity Source
  Mechanical Rotational Reference4 : fl_lib/Mechanical/Rotational Elements/Mechanical Rotational Reference
  Mechanical Rotational Reference8 : fl_lib/Mechanical/Rotational Elements/Mechanical Rotational Reference
  Reservoir (TL)1 : fl_lib/Thermal Liquid/Elements/Reservoir (TL)  pressure_spec=2  reservoir_pressure=0.1 MPa  reservoir_temperature=273.15+60 K  area=0.01 m^2
  Signal Editor : SignalEditorBlockLib/Signal Editor  FileName=Scenario2_Consumption.mat  ActiveScenario=Scenario1  ActiveSignal=Front Engine  IsBus=off  OutputBusObjectStr=Bus: BusObject  SampleTime=0  Interpolate=off  ZeroCross=off  OutputAfterFinalValue=Setting to zero  Unit=inherit  PreserveSignalName=on  ApplySigPropsToAllScenarios=on  ApplySigPropsToAllSignals=off
  Simulink-PS Converter : nesl_utility/Simulink-PS Converter  PhysicalDomain=network_engine_domain  SubClassName=ps_input  LeftPortType=input  RightPortType=output  PseudoPeriodic=off  Frequencies=[]  NoiseDistribution=none  NoiseParameters=[]  Unit=1  AffineConversion=off  FilteringAndDerivatives=provide  SimscapeFilterOrder=1  InputFilterTimeConstant=0.001  UdotUserProvided=0
  S : PMIOPort  Side=Right
  wires:
  Signal Editor/1 -> Simulink-PS Converter/1
  connections:
  Mechanical Rotational Reference8/LConn1 -- Ideal Angular Velocity Source2/RConn2
  Ideal Angular Velocity Source2/LConn1 -- Centrifugal Pump (TL)/RConn1
  Centrifugal Pump (TL)/RConn2 -- Mechanical Rotational Reference4/LConn1
  S/RConn1 -- Centrifugal Pump (TL)/LConn1
  Simulink-PS Converter/RConn1 -- Ideal Angular Velocity Source2/RConn1
  Centrifugal Pump (TL)/LConn2 -- Reservoir (TL)1/LConn1

== system AirCraft_Fuel_Distribution/Flow sensor  ==
  PS-Simulink Converter : nesl_utility/PS-Simulink Converter  PhysicalDomain=network_engine_domain  SubClassName=ps_output  LeftPortType=input  RightPortType=output  PseudoPeriodic=off  Frequencies=[]  Unit=inherit  AffineConversion=off
  Volumetric Flow Rate Sensor (TL) : fl_lib/Thermal Liquid/Sensors/Volumetric Flow Rate Sensor (TL)
      settings: InternalSimscapePortConfiguration="{\"Bottom\":[],\"Left\":[{\"id\":\"A\",\"label\":\"A\",\"type\":\"foundation.thermal_liquid.thermal_liquid\"}],\"Right\":[{\"id\":\"B\",\"label\":\"B\",\"type\":\"foundation.thermal_liquid.thermal_liquid\"},{\"id\":\"V\",\"label\":\"V\",\"type\":\"output\"}],\"Top\":[]}"
  A : PMIOPort  Side=Left
  B : PMIOPort  Port=2  Side=Right
  Out1 : Outport
  wires:
  PS-Simulink Converter/1 -> Out1/1
  connections:
  A/RConn1 -- Volumetric Flow Rate Sensor (TL)/LConn1
  B/RConn1 -- Volumetric Flow Rate Sensor (TL)/RConn1
  PS-Simulink Converter/LConn1 -- Volumetric Flow Rate Sensor (TL)/RConn2

== system AirCraft_Fuel_Distribution/Flow sensor 1 ==
  PS-Simulink Converter : nesl_utility/PS-Simulink Converter  PhysicalDomain=network_engine_domain  SubClassName=ps_output  LeftPortType=input  RightPortType=output  PseudoPeriodic=off  Frequencies=[]  Unit=inherit  AffineConversion=off
  Volumetric Flow Rate Sensor (TL) : fl_lib/Thermal Liquid/Sensors/Volumetric Flow Rate Sensor (TL)
      settings: InternalSimscapePortConfiguration="{\"Bottom\":[],\"Left\":[{\"id\":\"A\",\"label\":\"A\",\"type\":\"foundation.thermal_liquid.thermal_liquid\"}],\"Right\":[{\"id\":\"B\",\"label\":\"B\",\"type\":\"foundation.thermal_liquid.thermal_liquid\"},{\"id\":\"V\",\"label\":\"V\",\"type\":\"output\"}],\"Top\":[]}"
  A : PMIOPort  Side=Left
  B : PMIOPort  Port=2  Side=Right
  Out1 : Outport
  wires:
  PS-Simulink Converter/1 -> Out1/1
  connections:
  A/RConn1 -- Volumetric Flow Rate Sensor (TL)/LConn1
  B/RConn1 -- Volumetric Flow Rate Sensor (TL)/RConn1
  PS-Simulink Converter/LConn1 -- Volumetric Flow Rate Sensor (TL)/RConn2

== system AirCraft_Fuel_Distribution/Flow sensor 2 ==
  PS-Simulink Converter : nesl_utility/PS-Simulink Converter  PhysicalDomain=network_engine_domain  SubClassName=ps_output  LeftPortType=input  RightPortType=output  PseudoPeriodic=off  Frequencies=[]  Unit=inherit  AffineConversion=off
  Volumetric Flow Rate Sensor (TL) : fl_lib/Thermal Liquid/Sensors/Volumetric Flow Rate Sensor (TL)
      settings: InternalSimscapePortConfiguration="{\"Bottom\":[],\"Left\":[{\"id\":\"A\",\"label\":\"A\",\"type\":\"foundation.thermal_liquid.thermal_liquid\"}],\"Right\":[{\"id\":\"B\",\"label\":\"B\",\"type\":\"foundation.thermal_liquid.thermal_liquid\"},{\"id\":\"V\",\"label\":\"V\",\"type\":\"output\"}],\"Top\":[]}"
  A : PMIOPort  Side=Left
  B : PMIOPort  Port=2  Side=Right
  Out1 : Outport
  wires:
  PS-Simulink Converter/1 -> Out1/1
  connections:
  A/RConn1 -- Volumetric Flow Rate Sensor (TL)/LConn1
  B/RConn1 -- Volumetric Flow Rate Sensor (TL)/RConn1
  PS-Simulink Converter/LConn1 -- Volumetric Flow Rate Sensor (TL)/RConn2

== system AirCraft_Fuel_Distribution/Flow sensor 3 ==
  PS-Simulink Converter : nesl_utility/PS-Simulink Converter  PhysicalDomain=network_engine_domain  SubClassName=ps_output  LeftPortType=input  RightPortType=output  PseudoPeriodic=off  Frequencies=[]  Unit=inherit  AffineConversion=off
  Volumetric Flow Rate Sensor (TL) : fl_lib/Thermal Liquid/Sensors/Volumetric Flow Rate Sensor (TL)
      settings: InternalSimscapePortConfiguration="{\"Bottom\":[],\"Left\":[{\"id\":\"A\",\"label\":\"A\",\"type\":\"foundation.thermal_liquid.thermal_liquid\"}],\"Right\":[{\"id\":\"B\",\"label\":\"B\",\"type\":\"foundation.thermal_liquid.thermal_liquid\"},{\"id\":\"V\",\"label\":\"V\",\"type\":\"output\"}],\"Top\":[]}"
  A : PMIOPort  Side=Left
  B : PMIOPort  Port=2  Side=Right
  Out1 : Outport
  wires:
  PS-Simulink Converter/1 -> Out1/1
  connections:
  A/RConn1 -- Volumetric Flow Rate Sensor (TL)/LConn1
  B/RConn1 -- Volumetric Flow Rate Sensor (TL)/RConn1
  PS-Simulink Converter/LConn1 -- Volumetric Flow Rate Sensor (TL)/RConn2

== system AirCraft_Fuel_Distribution/Flow sensor 4 ==
  Display : Display
  PS-Simulink Converter : nesl_utility/PS-Simulink Converter  PhysicalDomain=network_engine_domain  SubClassName=ps_output  LeftPortType=input  RightPortType=output  PseudoPeriodic=off  Frequencies=[]  Unit=inherit  AffineConversion=off
  Volumetric Flow Rate Sensor (TL) : fl_lib/Thermal Liquid/Sensors/Volumetric Flow Rate Sensor (TL)
      settings: InternalSimscapePortConfiguration="{\"Bottom\":[],\"Left\":[{\"id\":\"A\",\"label\":\"A\",\"type\":\"foundation.thermal_liquid.thermal_liquid\"}],\"Right\":[{\"id\":\"B\",\"label\":\"B\",\"type\":\"foundation.thermal_liquid.thermal_liquid\"},{\"id\":\"V\",\"label\":\"V\",\"type\":\"output\"}],\"Top\":[]}"
  A : PMIOPort  Side=Left
  B : PMIOPort  Port=2  Side=Right
  Out1 : Outport
  wires:
  PS-Simulink Converter/1 -> Display/1, Out1/1
  connections:
  A/RConn1 -- Volumetric Flow Rate Sensor (TL)/LConn1
  B/RConn1 -- Volumetric Flow Rate Sensor (TL)/RConn1
  PS-Simulink Converter/LConn1 -- Volumetric Flow Rate Sensor (TL)/RConn2

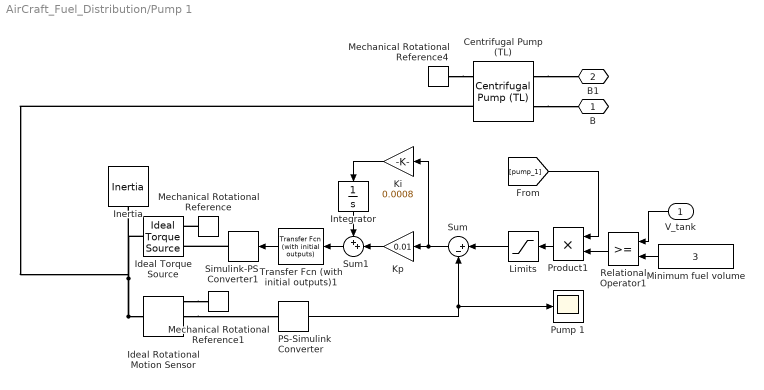
== system AirCraft_Fuel_Distribution/Pump 1 ==
  V_tank : Inport
  Centrifugal Pump (TL) : SimscapeFluids_lib/Thermal Liquid/Pumps & Motors/Centrifugal Pump (TL)  pump_parameterization=1  mech_orientation=1  flow_rate_1D_TLU=pump_wing(:,1) m^3/s  head_1D_TLU=pump_wing(:,2)./(9.81*rho_ref) m  power_1D_TLU=pump_wing(:,3) W  rho_ref_1D=rho_ref kg/m^3  omega_ref_1D=omega_ref rad/s  flow_rate_2D_TLU=[16.67, 23.33, 30, 40, 53.33, 60] lpm  omega_2D_TLU=[2450, 2800, 3150, 3500] rpm  head_2D_TLU=[25, 32.7, 42.5, 50; 24, 31.7, 41, 49; 22.7, 30.5, 39, 47.5; 20, 28, 36, 45; 15.7, 24, 32, 40; 12.5, 21, 29.5, 37.5] m  power_2D_TLU=[.28, .38, .5, .6; .31, .41, .55, .68; .33, .44, .6, .75; .36, .48, .65, .83; .38, .53, .72, .93; .39, .55, .75, .97] kW  rho_ref_2D=920 kg/m^3  omega_threshold=omega_threshold rad/s  area=area_pipe m^2  mdot_A_specify=off  mdot_A_priority=None  mdot_A=1 kg/s  mdot_A_nominal_specify=off  mdot_A_nominal_unit=kg/s  mdot_A_nominal_value=1
      settings: InternalSimscapePortConfiguration="{\"Bottom\":[],\"Left\":[{\"id\":\"A\",\"label\":\"A\",\"type\":\"foundation.thermal_liquid.thermal_liquid\"},{\"id\":\"B\",\"label\":\"B\",\"type\":\"foundation.thermal_liquid.thermal_liquid\"}],\"Right\":[{\"id\":\"R\",\"label\":\"R\",\"type\":\"foundation.mechanical.rotational.rotational\"},{\"id\":\"C\",\"label\":\"C\",\"type\":\"foundation.mechanical.rotational.rotational\"}],\"Top\":[]}"
  Ideal Rotational Motion Sensor : fl_lib/Mechanical/Mechanical Sensors/Ideal Rotational Motion Sensor  wrap_angle=simscape.enum.onoff.off  offset=0 rad
  Ideal Torque Source : fl_lib/Mechanical/Mechanical Sources/Ideal Torque Source
  Inertia : fl_lib/Mechanical/Rotational Elements/Inertia  inertia=0.005 kg*m^2  w_specify=on  w_priority=High  w=omega_min rev/s  w_nominal_specify=off  w_nominal_unit=rad/s  w_nominal_value=1  t_specify=off  t_priority=None  t=0 N*m  t_nominal_specify=off  t_nominal_unit=N*m  t_nominal_value=1
  Integrator : Integrator  LimitOutput=on  UpperSaturationLimit=1  LowerSaturationLimit=-1
  Ki : Gain  Gain=0.0008
  Kp : Gain  Gain=0.01
  Limits : Saturate  UpperLimit=210  LowerLimit=20
  Mechanical Rotational Reference : fl_lib/Mechanical/Rotational Elements/Mechanical Rotational Reference
  Mechanical Rotational Reference1 : fl_lib/Mechanical/Rotational Elements/Mechanical Rotational Reference
  Mechanical Rotational Reference4 : fl_lib/Mechanical/Rotational Elements/Mechanical Rotational Reference
  Minimum fuel volume : Constant  Value=3
  PS-Simulink Converter : nesl_utility/PS-Simulink Converter  PhysicalDomain=network_engine_domain  SubClassName=ps_output  LeftPortType=input  RightPortType=output  PseudoPeriodic=off  Frequencies=[]  Unit=rev/s  AffineConversion=off
  Product1 : Product  RndMeth=Zero
  Pump 1 : Scope
  Relational Operator1 : RelationalOperator  OutDataTypeStr=boolean  InputSameDT=off
  Simulink-PS Converter1 : nesl_utility/Simulink-PS Converter  PhysicalDomain=network_engine_domain  SubClassName=ps_input  LeftPortType=input  RightPortType=output  PseudoPeriodic=off  Frequencies=[]  NoiseDistribution=none  NoiseParameters=[]  Unit=N*m  AffineConversion=off  FilteringAndDerivatives=provide  SimscapeFilterOrder=1  InputFilterTimeConstant=0.001  UdotUserProvided=0
  Sum : Sum  Inputs=|+-
  Sum1 : Sum  Inputs=++|
  Transfer Fcn (with initial outputs)1 : simulink_extras/Additional Linear/Transfer Fcn (with initial outputs)  N=[1]  D=[mover_time_constant 1]  Y0=0  U0=0
  B : PMIOPort  Side=Left
  B1 : PMIOPort  Port=2  Side=Left
  wires:
  Product1/1 -> Limits/1
  Ki/1 -> Integrator/1
  Integrator/1 -> Sum1/1
  Kp/1 -> Sum1/2
  Transfer Fcn (with initial outputs)1/1 -> Simulink-PS Converter1/1
  Limits/1 -> Sum/1
  Sum1/1 -> Transfer Fcn (with initial outputs)1/1
  Minimum fuel volume/1 -> Relational Operator1/2
  Sum/1 -> Ki/1, Kp/1
  PS-Simulink Converter/1 -> Pump 1/1, Sum/2
  V_tank/1 -> Relational Operator1/1
  Relational Operator1/1 -> Product1/2
  [pump_1] -> Product1/1
  connections:
  Centrifugal Pump (TL)/LConn1 -- B/RConn1
  Centrifugal Pump (TL)/LConn2 -- B1/RConn1
  Mechanical Rotational Reference4/LConn1 -- Centrifugal Pump (TL)/RConn2
  Ideal Rotational Motion Sensor/LConn1 -- Centrifugal Pump (TL)/RConn1 -- Ideal Torque Source/LConn1 -- Inertia/LConn1
  Ideal Rotational Motion Sensor/RConn1 -- Mechanical Rotational Reference1/LConn1
  Mechanical Rotational Reference/LConn1 -- Ideal Torque Source/RConn2
  Simulink-PS Converter1/RConn1 -- Ideal Torque Source/RConn1
  Ideal Rotational Motion Sensor/RConn2 -- PS-Simulink Converter/LConn1

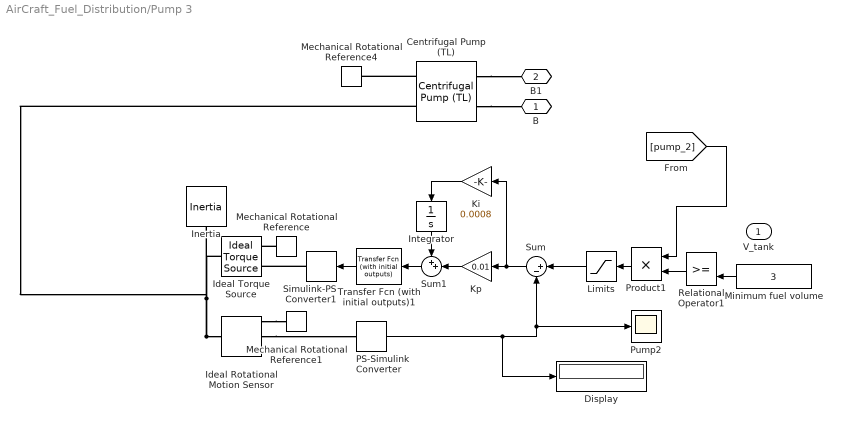
== system AirCraft_Fuel_Distribution/Pump 3 ==
  V_tank : Inport
  Centrifugal Pump (TL) : SimscapeFluids_lib/Thermal Liquid/Pumps & Motors/Centrifugal Pump (TL)  pump_parameterization=1  mech_orientation=1  flow_rate_1D_TLU=pump_wing(:,1) m^3/s  head_1D_TLU=pump_wing(:,2)./(9.81*rho_ref) m  power_1D_TLU=pump_wing(:,3) W  rho_ref_1D=rho_ref kg/m^3  omega_ref_1D=omega_ref rad/s  flow_rate_2D_TLU=[16.67, 23.33, 30, 40, 53.33, 60] lpm  omega_2D_TLU=[2450, 2800, 3150, 3500] rpm  head_2D_TLU=[25, 32.7, 42.5, 50; 24, 31.7, 41, 49; 22.7, 30.5, 39, 47.5; 20, 28, 36, 45; 15.7, 24, 32, 40; 12.5, 21, 29.5, 37.5] m  power_2D_TLU=[.28, .38, .5, .6; .31, .41, .55, .68; .33, .44, .6, .75; .36, .48, .65, .83; .38, .53, .72, .93; .39, .55, .75, .97] kW  rho_ref_2D=920 kg/m^3  omega_threshold=omega_threshold rad/s  area=area_pipe m^2  mdot_A_specify=off  mdot_A_priority=None  mdot_A=1 kg/s  mdot_A_nominal_specify=off  mdot_A_nominal_unit=kg/s  mdot_A_nominal_value=1
      settings: InternalSimscapePortConfiguration="{\"Bottom\":[],\"Left\":[{\"id\":\"A\",\"label\":\"A\",\"type\":\"foundation.thermal_liquid.thermal_liquid\"},{\"id\":\"B\",\"label\":\"B\",\"type\":\"foundation.thermal_liquid.thermal_liquid\"}],\"Right\":[{\"id\":\"R\",\"label\":\"R\",\"type\":\"foundation.mechanical.rotational.rotational\"},{\"id\":\"C\",\"label\":\"C\",\"type\":\"foundation.mechanical.rotational.rotational\"}],\"Top\":[]}"
  Display : Display
  Ideal Rotational Motion Sensor : fl_lib/Mechanical/Mechanical Sensors/Ideal Rotational Motion Sensor  wrap_angle=simscape.enum.onoff.off  offset=0 rad
  Ideal Torque Source : fl_lib/Mechanical/Mechanical Sources/Ideal Torque Source
  Inertia : fl_lib/Mechanical/Rotational Elements/Inertia  inertia=0.005 kg*m^2  w_specify=on  w_priority=High  w=omega_min rev/s  w_nominal_specify=off  w_nominal_unit=rad/s  w_nominal_value=1  t_specify=off  t_priority=None  t=0 N*m  t_nominal_specify=off  t_nominal_unit=N*m  t_nominal_value=1
  Integrator : Integrator  LimitOutput=on  UpperSaturationLimit=1  LowerSaturationLimit=-1
  Ki : Gain  Gain=0.0008
  Kp : Gain  Gain=0.01
  Limits : Saturate  UpperLimit=220  LowerLimit=20
  Mechanical Rotational Reference : fl_lib/Mechanical/Rotational Elements/Mechanical Rotational Reference
  Mechanical Rotational Reference1 : fl_lib/Mechanical/Rotational Elements/Mechanical Rotational Reference
  Mechanical Rotational Reference4 : fl_lib/Mechanical/Rotational Elements/Mechanical Rotational Reference
  Minimum fuel volume : Constant  Value=3
  PS-Simulink Converter : nesl_utility/PS-Simulink Converter  PhysicalDomain=network_engine_domain  SubClassName=ps_output  LeftPortType=input  RightPortType=output  PseudoPeriodic=off  Frequencies=[]  Unit=rev/s  AffineConversion=off
  Product1 : Product  RndMeth=Zero
  Pump2 : Scope
  Relational Operator1 : RelationalOperator  OutDataTypeStr=boolean  InputSameDT=off
  Simulink-PS Converter1 : nesl_utility/Simulink-PS Converter  PhysicalDomain=network_engine_domain  SubClassName=ps_input  LeftPortType=input  RightPortType=output  PseudoPeriodic=off  Frequencies=[]  NoiseDistribution=none  NoiseParameters=[]  Unit=N*m  AffineConversion=off  FilteringAndDerivatives=provide  SimscapeFilterOrder=1  InputFilterTimeConstant=0.001  UdotUserProvided=0
  Sum : Sum  Inputs=|+-
  Sum1 : Sum  Inputs=++|
  Transfer Fcn (with initial outputs)1 : simulink_extras/Additional Linear/Transfer Fcn (with initial outputs)  N=[1]  D=[mover_time_constant 1]  Y0=0  U0=0
  B : PMIOPort  Side=Left
  B1 : PMIOPort  Port=2  Side=Left
  wires:
  Product1/1 -> Limits/1
  Ki/1 -> Integrator/1
  Integrator/1 -> Sum1/1
  Kp/1 -> Sum1/2
  Transfer Fcn (with initial outputs)1/1 -> Simulink-PS Converter1/1
  Limits/1 -> Sum/1
  Sum1/1 -> Transfer Fcn (with initial outputs)1/1
  Minimum fuel volume/1 -> Relational Operator1/2
  Sum/1 -> Ki/1, Kp/1
  PS-Simulink Converter/1 -> Display/1, Pump2/1, Sum/2
  Relational Operator1/1 -> Product1/2
  [pump_2] -> Product1/1
  connections:
  Centrifugal Pump (TL)/RConn2 -- Mechanical Rotational Reference4/LConn1
  Centrifugal Pump (TL)/LConn2 -- B1/RConn1
  Centrifugal Pump (TL)/LConn1 -- B/RConn1
  Ideal Rotational Motion Sensor/LConn1 -- Centrifugal Pump (TL)/RConn1 -- Ideal Torque Source/LConn1 -- Inertia/LConn1
  Ideal Rotational Motion Sensor/RConn1 -- Mechanical Rotational Reference1/LConn1
  Mechanical Rotational Reference/LConn1 -- Ideal Torque Source/RConn2
  Simulink-PS Converter1/RConn1 -- Ideal Torque Source/RConn1
  Ideal Rotational Motion Sensor/RConn2 -- PS-Simulink Converter/LConn1

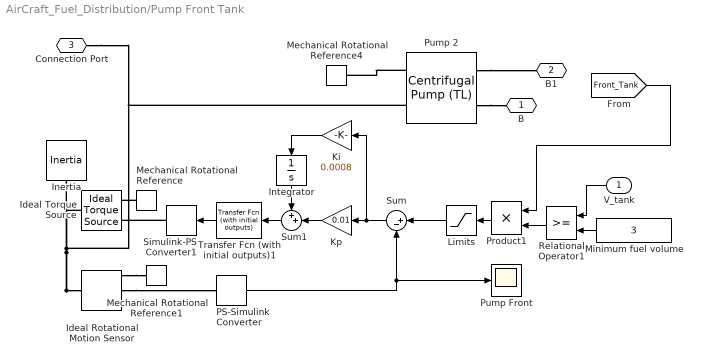
== system AirCraft_Fuel_Distribution/Pump Front Tank  ==
  V_tank : Inport
  Ideal Rotational Motion Sensor : fl_lib/Mechanical/Mechanical Sensors/Ideal Rotational Motion Sensor  wrap_angle=simscape.enum.onoff.off  offset=0 rad
  Ideal Torque Source : fl_lib/Mechanical/Mechanical Sources/Ideal Torque Source
  Inertia : fl_lib/Mechanical/Rotational Elements/Inertia  inertia=0.005 kg*m^2  w_specify=on  w_priority=High  w=omega_min rev/s  w_nominal_specify=off  w_nominal_unit=rad/s  w_nominal_value=1  t_specify=off  t_priority=None  t=0 N*m  t_nominal_specify=off  t_nominal_unit=N*m  t_nominal_value=1
  Integrator : Integrator  LimitOutput=on  UpperSaturationLimit=1  LowerSaturationLimit=-1
  Ki : Gain  Gain=0.0008
  Kp : Gain  Gain=0.01
  Limits : Saturate  UpperLimit=250  LowerLimit=20
  Mechanical Rotational Reference : fl_lib/Mechanical/Rotational Elements/Mechanical Rotational Reference
  Mechanical Rotational Reference1 : fl_lib/Mechanical/Rotational Elements/Mechanical Rotational Reference
  Mechanical Rotational Reference4 : fl_lib/Mechanical/Rotational Elements/Mechanical Rotational Reference
  Minimum fuel volume : Constant  Value=3
  PS-Simulink Converter : nesl_utility/PS-Simulink Converter  PhysicalDomain=network_engine_domain  SubClassName=ps_output  LeftPortType=input  RightPortType=output  PseudoPeriodic=off  Frequencies=[]  Unit=rev/s  AffineConversion=off
  Product1 : Product  RndMeth=Zero
  Pump 2 : SimscapeFluids_lib/Thermal Liquid/Pumps & Motors/Centrifugal Pump (TL)  pump_parameterization=1  mech_orientation=1  flow_rate_1D_TLU=pump_wing(:,1) m^3/s  head_1D_TLU=pump_wing(:,2)./(9.81*rho_ref) m  power_1D_TLU=pump_wing(:,3) W  rho_ref_1D=rho_ref kg/m^3  omega_ref_1D=omega_ref rev/s  flow_rate_2D_TLU=[16.67, 23.33, 30, 40, 53.33, 60] lpm  omega_2D_TLU=[2450, 2800, 3150, 3500] rpm  head_2D_TLU=[25, 32.7, 42.5, 50; 24, 31.7, 41, 49; 22.7, 30.5, 39, 47.5; 20, 28, 36, 45; 15.7, 24, 32, 40; 12.5, 21, 29.5, 37.5] m  power_2D_TLU=[.28, .38, .5, .6; .31, .41, .55, .68; .33, .44, .6, .75; .36, .48, .65, .83; .38, .53, .72, .93; .39, .55, .75, .97] W  rho_ref_2D=920 kg/m^3  omega_threshold=omega_threshold rad/s  area=area_pipe m^2  mdot_A_specify=off  mdot_A_priority=None  mdot_A=1 kg/s  mdot_A_nominal_specify=off  mdot_A_nominal_unit=kg/s  mdot_A_nominal_value=1
      settings: InternalSimscapePortConfiguration="{\"Bottom\":[],\"Left\":[{\"id\":\"A\",\"label\":\"A\",\"type\":\"foundation.thermal_liquid.thermal_liquid\"},{\"id\":\"B\",\"label\":\"B\",\"type\":\"foundation.thermal_liquid.thermal_liquid\"}],\"Right\":[{\"id\":\"R\",\"label\":\"R\",\"type\":\"foundation.mechanical.rotational.rotational\"},{\"id\":\"C\",\"label\":\"C\",\"type\":\"foundation.mechanical.rotational.rotational\"}],\"Top\":[]}"
  "Pump Front " : Scope
  Relational Operator1 : RelationalOperator  OutDataTypeStr=boolean  InputSameDT=off
  Simulink-PS Converter1 : nesl_utility/Simulink-PS Converter  PhysicalDomain=network_engine_domain  SubClassName=ps_input  LeftPortType=input  RightPortType=output  PseudoPeriodic=off  Frequencies=[]  NoiseDistribution=none  NoiseParameters=[]  Unit=N*m  AffineConversion=off  FilteringAndDerivatives=provide  SimscapeFilterOrder=1  InputFilterTimeConstant=0.001  UdotUserProvided=0
  Sum : Sum  Inputs=|+-
  Sum1 : Sum  Inputs=++|
  Transfer Fcn (with initial outputs)1 : simulink_extras/Additional Linear/Transfer Fcn (with initial outputs)  N=[1]  D=[0.2 1]  Y0=0  U0=0
  B : PMIOPort  Side=Left
  B1 : PMIOPort  Port=2  Side=Left
  Connection Port : PMIOPort  Port=3  Side=Left
  wires:
  Product1/1 -> Limits/1
  Ki/1 -> Integrator/1
  Integrator/1 -> Sum1/1
  Kp/1 -> Sum1/2
  Transfer Fcn (with initial outputs)1/1 -> Simulink-PS Converter1/1
  Limits/1 -> Sum/1
  Sum1/1 -> Transfer Fcn (with initial outputs)1/1
  Minimum fuel volume/1 -> Relational Operator1/2
  Sum/1 -> Ki/1, Kp/1
  PS-Simulink Converter/1 -> Sum/2, "Pump Front "/1
  V_tank/1 -> Relational Operator1/1
  Relational Operator1/1 -> Product1/2
  [Front_Tank] -> Product1/1
  connections:
  Pump 2/RConn2 -- Mechanical Rotational Reference4/LConn1
  Ideal Rotational Motion Sensor/LConn1 -- Connection Port/RConn1 -- Pump 2/RConn1 -- Ideal Torque Source/LConn1 -- Inertia/LConn1
  Ideal Rotational Motion Sensor/RConn1 -- Mechanical Rotational Reference1/LConn1
  Mechanical Rotational Reference/LConn1 -- Ideal Torque Source/RConn2
  Simulink-PS Converter1/RConn1 -- Ideal Torque Source/RConn1
  Ideal Rotational Motion Sensor/RConn2 -- PS-Simulink Converter/LConn1
  Pump 2/LConn2 -- B1/RConn1
  Pump 2/LConn1 -- B/RConn1
